simulink library "propertySpecificationLib"  (Simulink 7.6)
settings: Solver=FixedStepDiscrete  StartTime=0.0  StopTime=10.0  FixedStep=Auto  RelTol=1e-3
undefined symbols (not defined in the file or in its folder): sldvsubsys
libraries: sldvlib x4
settings Model: Creator=itoy  LastModifiedBy=itoy

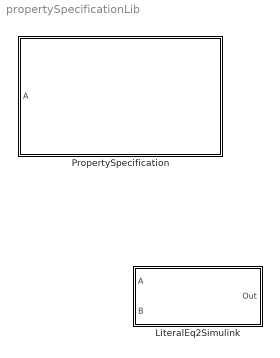
== system propertySpecificationLib ==
  LiteralEq2Simulink : Subsystem  Tag=CustomScope  mask(Equation2Simulink block){InputVar=A,B, ParamVar=, VerifEq=A==B}
      mask prompts: InputVar "“ü—Í•Ï?”"; ParamVar "ƒpƒ‰ƒ??[ƒ^•Ï?”"; VerifEq "ŒŸ?¸Ž®"
      mask help: Equation2Simulink block
      mask init:
      | Equation2Simulink(VerifEq,gcb,InputVar,ParamVar);
      mask Display: disp(VerifEq)
  PropertySpecification : Subsystem  Tag=VerificationSubsystem  DisableCoverage=on  LoadFcn=sldvsubsys('check')  TreatAsAtomicUnit=on  SimViewingDevice=on  mask(VerificationSubsystem){}
      mask help: Property Specification Block
      mask init:
      | sldvsubsys('maskInit');
      settings: OpenFcn=PropertySpecificationUI('Block',gcb)
      settings: CopyFcn=|
      | sldvsubsys('copy');
      |  set_param(gcb,'LinkStatus','none')
      settings: PreSaveFcn=|
      | set_param(gcb,'SimViewingDevice','on');
      | sldvsubsys('check');
      mask Help: helpview(fullfile(docroot,'toolbox','sldv','sldv.map'),'verificationsubsystem')
      mask Display: image(imread('sldvicon_versubsys.png','BackGroundColor',[1 1 1]),'center');

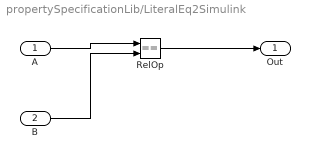
== system propertySpecificationLib/LiteralEq2Simulink ==
  A : Inport
  B : Inport  Port=2
  RelOp : RelationalOperator  Operator===  InputSameDT=on
  Out : Outport
  wires:
  A/1 -> RelOp/1
  RelOp/1 -> Out/1
  B/1 -> RelOp/2

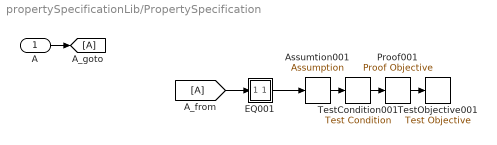
== system propertySpecificationLib/PropertySpecification ==
  A : Inport
  Assumtion001 : sldvlib/Assumption  SystemSampleTime=-1  enabled=off  customAVTBlockType=Assumption  intervals=true  initial=off  dispValues=on  outEnabled=on
      settings: AttributesFormatString=%<intervals>
  EQ001 : Subsystem  Tag=CustomScope  mask(Equation2Simulink block){InputVar=A, ParamVar=, VerifEq=A==1}
      mask prompts: InputVar "“ü—Í•Ï?”"; ParamVar "ƒpƒ‰ƒ??[ƒ^•Ï?”"; VerifEq "ŒŸ?¸Ž®"
      mask help: Equation2Simulink block
      mask init:
      | Equation2Simulink(VerifEq,gcb,InputVar,ParamVar);
      mask Display: disp(VerifEq)
  Proof001 : sldvlib/Proof Objective  SystemSampleTime=-1  enabled=on  customAVTBlockType=Proof Objective  intervals=true  dispValues=on  outEnabled=on  enableStopSim=off
      settings: AttributesFormatString=%<intervals>
  TestCondition001 : sldvlib/Test Condition  SystemSampleTime=-1  enabled=off  customAVTBlockType=Test Condition  intervals=true  initial=off  dispValues=on  outEnabled=on
      settings: AttributesFormatString=%<intervals>
  TestObjective001 : sldvlib/Test Objective  SystemSampleTime=-1  enabled=on  customAVTBlockType=Test Objective  intervals=true  dispValues=on  outEnabled=off
      settings: AttributesFormatString=%<intervals>
  wires:
  A/1 -> [A]
  [A] -> EQ001/1(A)
  Proof001/1 -> TestObjective001/1
  TestCondition001/1 -> Proof001/1
  Assumtion001/1 -> TestCondition001/1
  EQ001/1(Out) -> Assumtion001/1

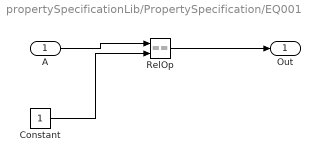
== system propertySpecificationLib/PropertySpecification/EQ001 ==
  A : Inport
  Constant : Constant  OutDataTypeStr=Inherit: Inherit via back propagation
  RelOp : RelationalOperator  Operator===  InputSameDT=on
  Out : Outport
  wires:
  Constant/1 -> RelOp/2
  RelOp/1 -> Out/1
  A/1 -> RelOp/1
